simulink model "nieLiniowyModelWachadlaOdwruconego_v2"  (R2017a)
settings: Solver=VariableStepAuto  StartTime=0.0  StopTime=100  MaxStep=0.1  MinStep=0.001  RelTol=1e-5
undefined symbols (not defined in the file or in its folder): K0, K30
libraries: fuzblock x1
settings Model: Creator=Szwank  LastModifiedBy=Szwank

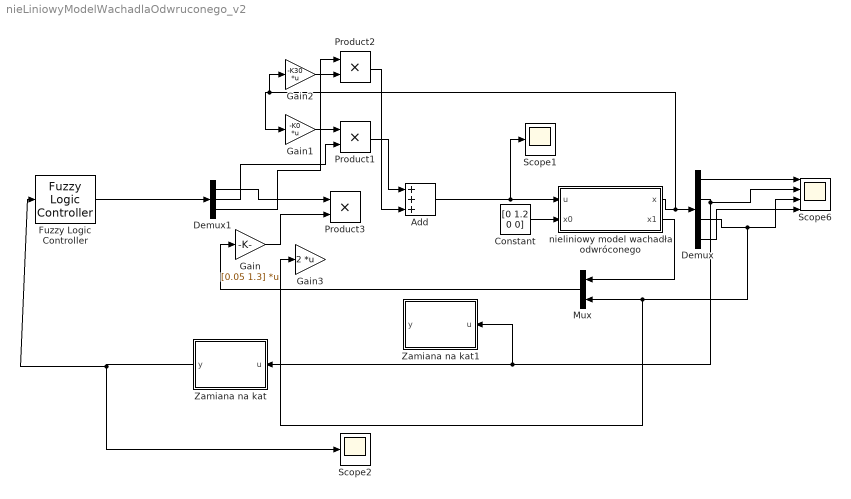
== system nieLiniowyModelWachadlaOdwruconego_v2 ==
  " nieliniowy model wachadła odwróconego" : Subsystem
  Add : Sum  Inputs=+++
  Constant : Constant  Value=[0 1.2 0 0]
  Demux : Demux
  Demux1 : Demux  Outputs=3
  Fuzzy Logic Controller : fuzblock/Fuzzy Logic  Controller  fis='RegulatorRozmyty_v2.fis'
  Gain : Gain  Gain=[0.05 1.3]  Multiplication=Matrix(K*u)
  Gain1 : Gain  Gain=-K0  Multiplication=Matrix(K*u)
  Gain2 : Gain  Gain=-K30  Multiplication=Matrix(K*u)
  Gain3 : Gain  Gain=2  Multiplication=Matrix(K*u)
  Mux : Mux  Inputs=2
  Product1 : Product
  Product2 : Product
  Product3 : Product
  Scope1 : Scope
  Scope2 : Scope
  Scope6 : Scope  NumInputPorts=4
  Zamiana na kat : MATLAB Function  TreatAsAtomicUnit=on
  Zamiana na kat1 : MATLAB Function  TreatAsAtomicUnit=on
  wires:
  Constant/1 -> " nieliniowy model wachadła odwróconego"/2(x0)
  " nieliniowy model wachadła odwróconego"/1(x) -> Gain2/1, Gain1/1, Demux/1
  Demux/1 -> Scope6/1
  Demux/4 -> Scope6/4
  Add/1 -> Scope1/1, " nieliniowy model wachadła odwróconego"/1(u)
  Mux/1 -> Gain/1
  Demux/2 -> Scope6/2, Zamiana na kat/1(u), Zamiana na kat1/1(u)
  Zamiana na kat/1(y) -> Fuzzy Logic Controller/1, Scope2/1
  Gain1/1 -> Product1/1
  Demux1/2 -> Product1/2
  Demux1/1 -> Product3/1
  Product1/1 -> Add/1
  Fuzzy Logic Controller/1 -> Demux1/1
  Gain2/1 -> Product2/2
  Demux1/3 -> Product2/1
  Product2/1 -> Add/3
  Demux/3 -> Gain3/1, Mux/2, Scope6/3
  " nieliniowy model wachadła odwróconego"/2(x1) -> Mux/1
  Gain/1 -> Product3/2

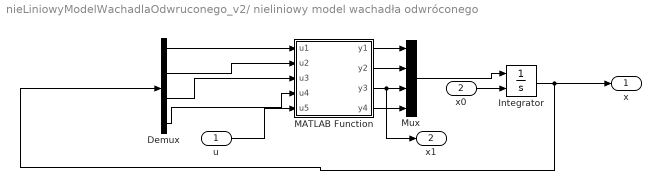
== system nieLiniowyModelWachadlaOdwruconego_v2/ nieliniowy model wachadła odwróconego ==
  u : Inport
  x0 : Inport  Port=2
  Demux : Demux
  Integrator : Integrator  InitialConditionSource=external  InitialCondition=[0 pi/6 0 0]
  MATLAB Function : MATLAB Function  TreatAsAtomicUnit=on
  Mux : Mux
  x : Outport
  x1 : Outport  Port=2
  wires:
  Mux/1 -> Integrator/1
  Demux/1 -> MATLAB Function/1(u1)
  MATLAB Function/2(y2) -> Mux/2
  Demux/4 -> MATLAB Function/4(u4)
  MATLAB Function/4(y4) -> Mux/4
  Integrator/1 -> x/1, Demux/1
  MATLAB Function/1(y1) -> Mux/1
  Demux/3 -> MATLAB Function/3(u3)
  MATLAB Function/3(y3) -> x1/1, Mux/3
  Demux/2 -> MATLAB Function/2(u2)
  u/1 -> MATLAB Function/5(u5)
  x0/1 -> Integrator/2

== matlab function nieLiniowyModelWachadlaOdwruconego_v2/ nieliniowy model wachadła odwróconego/MATLAB Function ==
  data: u1 input; y1 output; u2 input; u3 input; u4 input; u5 input; y2 output; y3 output; y4 output
function [y1,y2,y3,y4] = fcn(u1,u2,u3,u4,u5)
%Dane obiektu
%% Motor
Rm = 3.3; % ohms, Motor armature resistance 
Kt = 0.0280; % N.m, Motor torque constant
Km = 0.0280; % V/(rad/s), Motor back-emf constant (same as Ktin SI units)
Jm = 9.64e-6; % kg.m2, Moment of inertia of motor rotor. 
Jeq = 1.23e-4; % kg.m2, Equivalent moment of inertia about motor shaft pivot axis.
%% Pendulum Arm:
Marm = 0.0280; % kg, Mass of the arm.
r = 0.0826; % m, Length of arm pivot to pendulum pivot.
Beq = 0.001; % N.m/(rad/s), Arm viscous damping. 
%% Pendulum Link:
Mp = 0.0270; % kg, Mass of the pendulum link and weight combined.
Lp = 0.191; % m, Total length of pendulum.
lp = 0.153; % m, Length of pendulum center of mass from pivot.
Jp = 1.20e-4; % kg.m2, Pendulum moment of inertia about its pivot axis.
Bp = 0; % N.m/(rad/s), Pendulum viscous damping.
%% Pulse-Width Modulated Amplifier:
Vmax = 24; % V, PWM amplifier maximum output voltage
PWM = 5; % A, amplifier maximum output current
Kw = 2.3; % V/V, PWM amplifier gain
%% Stałe
m = Mp;
g = 9.80665;
a = Jeq + m * r^2;
b = m * lp * r;
e = m*lp^2 + Jp;
f = m*g*lp;
c = Km*Kw/Rm;
d = (Km*Kt+Beq*Rm)/Rm;
%%

y1 = u3;
y2 = u4;
y3 = 1/(1-(b^2/(a*e))*cos(u2)^2)*(1/a)*(b*f/e*sin(u2)*cos(u2)-b*u4^2*sin(u2)+u5*c-d*u3);
y4 = 1/(1-(b^2/(a*e))*cos(u2)^2)*(1/e)*(b/a*cos(u2)*(-b*u4^2*sin(u2)+c*u5-d*u3)+f*sin(u2));

== matlab function nieLiniowyModelWachadlaOdwruconego_v2/Zamiana na kat1 ==
  data: u input; y output
function y = fcn(u)


if(u>2*pi||u<-2*pi)
    
u=rem(u,2*pi);

end
y = u;

== matlab function nieLiniowyModelWachadlaOdwruconego_v2/Zamiana na kat ==
  data: u input; y output
function y = fcn(u)

u=rem(u,2*pi);


if(u>0)
    if(u>pi)
        u=-pi+rem(u,pi);
    end
end

if(u<0)
    if(u<-pi)
        u=pi+rem(u,pi);
    end
end
y = u;
